simulink model "gm_fil_videosharp_sim"  (R2019a)
settings: Solver=FixedStepDiscrete  StartTime=0.0  StopTime=0.21  RelTol=1e-3
InitFcn:
  | filter = fi(fspecial('unsharp'),1,16,12);
  | 
  | % video size excluding the blanking periods
  | fileName = get_param('fil_videosharp_sim/From Multimedia File',  'inputFilename');
  | x=mmfileinfo(fileName);
  | v = x.Video ;
  | H = v.Height;
  | W = v.Width;
  | %H = 176;
  | %W = 240;
  | activeVideoSize = [H W];
  | 
  | % horizontal and vertical blanking
  | hBlanking = 0;
  | vBlanking = 0;
undefined symbols (not defined in the file or in its folder): fspecial, gcbh, NumBits1, NumBits2, Rec, SDTV, Slope1, Slope2
libraries: simulink x19, visionconversions x3, dspsigattribs x3, dspbuff3 x3, hdlsllib x3, visionsinks x1, dspvision x1, simulink_need_slupdate x1
(part 1 of 3)
settings Model: FPTRunName=Active  SimulationMode=accelerator  ExtModeAutoUpdateStatusClock=off  Creator=wjachimc  LastModifiedBy=rbhar
settings DataIOCC: LimitDataPoints=on  SaveFormat=Structure  SignalLoggingSaveFormat=ModelDataLogs  SaveOutput=off  InspectSignalLogs=on  SaveTime=off  ReturnWorkspaceOutputs=off
settings OptimizationCC: BlockReduction=off  ConditionallyExecuteInputs=off  ExpressionDepthLimit=2147483647  InitFltsAndDblsToZero=on  EfficientMapNaN2IntZero=off  LifeSpan=inf
settings DebuggingCC: UnderspecifiedInitializationDetection=Classic  MergeDetectMultiDrivingBlocksExec=none  InheritedTsInSrcMsg=none  SingleTaskRateTransMsg=error  IntegerOverflowMsg=none  FcnCallInpInsideContextMsg=warning  StateNameClashWarn=warning  PregeneratedLibrarySubsystemCodeDiagnostic=none  SFUnexpectedBacktrackingDiag=warning  SFNoUnconditionalDefaultTransitionDiag=warning  SFExecutionAtInitializationDiag=none  IntegerSaturationMsg=none  ArithmeticOperatorsInVariantConditions=warning
settings HardwareCC: ProdBitPerPointer=32  ProdBitPerSizeT=32  ProdBitPerPtrDiffT=32  ProdLargestAtomicFloat=None  ProdIntDivRoundTo=Undefined  ProdEndianess=Unspecified  ProdWordSize=32  ProdHWDeviceType=ASIC/FPGA->ASIC/FPGA  TargetBitPerPointer=64  TargetBitPerSizeT=64  TargetBitPerPtrDiffT=64  TargetLongLongMode=on  TargetIntDivRoundTo=Zero  TargetEndianess=LittleEndian  TargetWordSize=64  TargetHWDeviceType=MATLAB Host  ProdEqTarget=off
settings ModelReferenceCC: PropagateSignalLabelsOutOfModel=off
settings SFSimCC: SimUseLocalCustomCode=off  SimParseCustomCode=off
settings RTWCC: RTWUseLocalCustomCode=off
settings CodeAppCC: StateflowObjectComments=on
settings GRTTargetCC: TargetLangStandard=C89/C90 (ANSI)  GeneratePreprocessorConditionals=Disable all  CombineOutputUpdateFcns=off  GRTInterface=on
settings ConfigComp: CovMetricSettings=dw  CovHtmlReporting=on  CovSaveCumulativeToWorkspaceVar=on  CovSaveSingleToWorkspaceVar=on  CovExternalEMLEnable=off

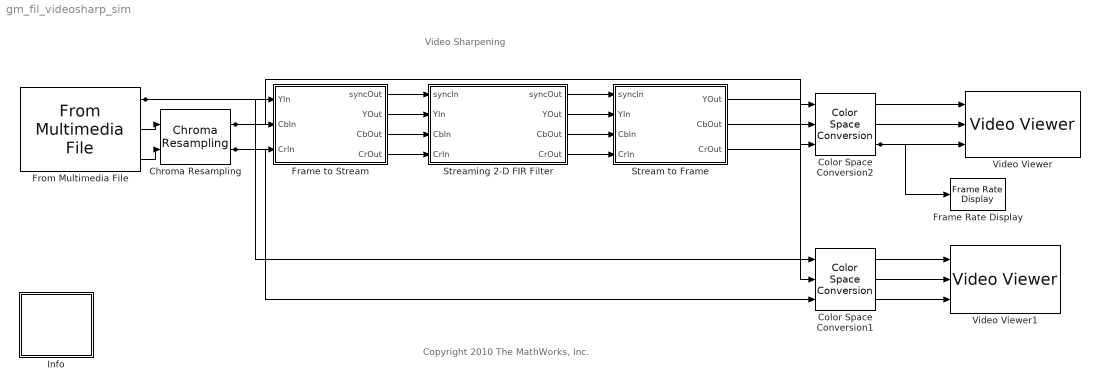
== system gm_fil_videosharp_sim ==
  note: Copyright 2010 The MathWorks, Inc.
  note: Video Sharpening
  Chroma Resampling : visionconversions/Chroma Resampling  resampling=4:2:2 to 4:4:4  interpolation=linear  antialiasing=Default  hcoeff=[0.2 0.6 0.2]  vcoeff=[0.5 0.5]  isInputTransposed=off
      settings: SourceProductName=Computer Vision System Toolbox  SourceProductBaseCode=VP
  Color Space Conversion1 : visionconversions/Color Space  Conversion  conversion=Obsolete  conversionActive=Y'CbCr to R'G'B'  wp_str=D65  rec=Rec. 601 (SDTV)  sys=1125/60/2:1  imagePorts=Separate color signals
      settings: SourceProductName=Computer Vision System Toolbox
  Color Space Conversion2 : visionconversions/Color Space  Conversion  conversion=Obsolete  conversionActive=Y'CbCr to R'G'B'  wp_str=D65  rec=Rec. 601 (SDTV)  sys=1125/60/2:1  imagePorts=Separate color signals
      settings: SourceProductName=Computer Vision System Toolbox
  Frame Rate Display : visionsinks/Frame Rate Display  UpdateRate=3
      settings: SourceProductName=Computer Vision System Toolbox  SourceProductBaseCode=VP
  Frame to Stream : Subsystem  mask(Frame to Stream){hBlanking=hBlanking, vBlanking=vBlanking, isInputRowMajor=off}
      mask prompts: hBlanking "Horizontal blanking:"; vBlanking "Vertical blanking:"; isInputRowMajor "Input image is transposed"
      mask help:
      | This blocks converts a full frame video input into a pixel stream with additional synchronization signals.
      |
      | The specified amount, in pixels, of horizontal blanking is prepended to the left of the video frame while the amount of vertical blanking is appended to the bottom of the video frame.
      mask Display: disp(sprintf('%s\n%s','Frame to', 'Stream'));
  From Multimedia File : dspvision/From Multimedia File  inputFilename=fil_cat.avi  readRange=[1 Inf]  loop=on  numPlays=inf  outputStreams=Video only  videoDataType=uint8  audioDataType=int16  inheritSampleTime=on  userDefinedSampleTime=1  noAudioOutput=off  isIntensityVideo=off  fourcc=YCbCr 4:2:2  colorVideoFormat=Separate color signals  outputEOF=off  dataOrg=Column-major  audioFrameSize=1838  computeAudioFrameSize=off  outSamplingMode=Frame based
      settings: SourceProductBaseCode=VP
  Info : Subsystem  mask(Info){}
      settings: OpenFcn=showdemo('fil_videosharp_sim');
      mask Display: image(imread('fil_demo_info.bmp','bmp'))
  Stream to Frame : Subsystem  mask(Stream to Frame){frameSize=activeVideoSize}
      mask prompts: frameSize "Frame size"
      mask help: Converts stream of pixels into a full frame video based on the corresponding synchronization signals.
      mask Display: disp(sprintf('%s\n%s', 'Stream to', 'Frame'));
  Streaming 2-D FIR Filter : Subsystem  mask(Streaming 2-D FIR Filter){frame_size=activeVideoSize, FILTCOEFF=fi(fspecial('gaussian',[3,3],0.5), 1, 16, 12), PADDING=Replicate, PADVAL=0}
      mask prompts: frame_size "Frame size:"; FILTCOEFF "Filter Coefficient:"; PADDING "Padding Options"; PADVAL "Constant value for padding:"
      mask help: 2-D FIR suitable for FPGA .
      mask init:
      | blkh=gcbh;
      | main_blk = [get(blkh, 'parent'), '/', get(blkh, 'name')];
      | sub_blk = [main_blk, '/', 'Make Neighborhood'];
      | main_value = get_param(main_blk,'PADDING');
      | set_param(sub_blk,'PADDING',main_value);
      | 
      | main_value = get_param(main_blk,'PADVAL');
      | set_param(sub_blk,'PADVAL',main_value);
      mask TypeOptions PADDING: Constant | Replicate | Symmetric
      mask Callback PADDING:
      | maskStr = get_param(gcb,'MaskValues');
      | maskvisi = get_param(gcb,'MaskVisibilities');
      | maskenebles = get_param(gcb,'MaskEnables');
      | if (strcmp(maskStr{3},'Constant') )
      |     maskvisi{4,1}='on';
      | else
      |     maskvisi{4,1}='off';
      | end
      | set_param(gcb,'MaskValues',maskStr);
      | set_param(gcb,'MaskVisibilities',maskvisi);
      | set_param(gcb,'MaskEnables',maskenebles)
      mask Display: disp(sprintf('%s\n%s', 'Streaming', '2-D FIR Filter'));
  Video Viewer : VideoViewer  imagePorts=separate color signals  FigPos=[435 661 410 300]
  Video Viewer1 : VideoViewer  imagePorts=separate color signals  FigPos=[436 659 408 297]
  wires:
  Streaming 2-D FIR Filter/4(CrOut) -> Stream to Frame/4(CrIn)
  Streaming 2-D FIR Filter/3(CbOut) -> Stream to Frame/3(CbIn)
  Frame to Stream/4(CrOut) -> Streaming 2-D FIR Filter/4(CrIn)
  Frame to Stream/3(CbOut) -> Streaming 2-D FIR Filter/3(CbIn)
  Chroma Resampling/2 -> Color Space Conversion1/3, Frame to Stream/3(CrIn)
  Chroma Resampling/1 -> Color Space Conversion1/2, Frame to Stream/2(CbIn)
  From Multimedia File/3 -> Chroma Resampling/2
  From Multimedia File/2 -> Chroma Resampling/1
  Color Space Conversion1/3 -> Video Viewer1/3
  Color Space Conversion1/2 -> Video Viewer1/2
  Color Space Conversion1/1 -> Video Viewer1/1
  Stream to Frame/3(CrOut) -> Color Space Conversion2/3
  Stream to Frame/2(CbOut) -> Color Space Conversion2/2
  Stream to Frame/1(YOut) -> Color Space Conversion2/1
  Color Space Conversion2/3 -> Video Viewer/3, Frame Rate Display/1
  Color Space Conversion2/2 -> Video Viewer/2
  Color Space Conversion2/1 -> Video Viewer/1
  Frame to Stream/2(YOut) -> Streaming 2-D FIR Filter/2(YIn)
  Frame to Stream/1(syncOut) -> Streaming 2-D FIR Filter/1(syncIn)
  Streaming 2-D FIR Filter/2(YOut) -> Stream to Frame/2(YIn)
  Streaming 2-D FIR Filter/1(syncOut) -> Stream to Frame/1(syncIn)
  From Multimedia File/1 -> Color Space Conversion1/1, Frame to Stream/1(YIn)

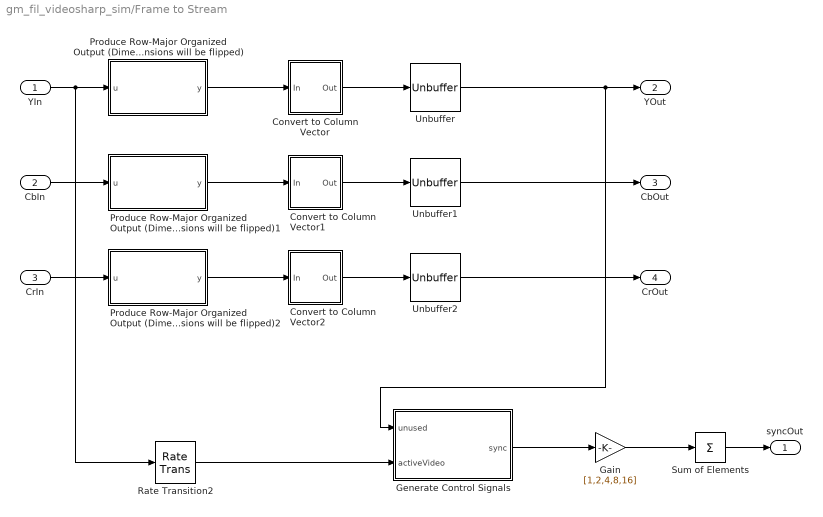
== system gm_fil_videosharp_sim/Frame to Stream ==
  YIn : Inport
  CbIn : Inport  Port=2
  CrIn : Inport  Port=3
  Convert to Column Vector : Subsystem
  Convert to Column Vector1 : Subsystem
  Convert to Column Vector2 : Subsystem
  Gain : Gain  Gain=[1,2,4,8,16]  ParamDataTypeStr=fixdt(0,5,0)  OutDataTypeStr=fixdt(0,5,0)
  Generate Control Signals : MATLAB Function  TreatAsAtomicUnit=on
  Produce Row-Major Organized Output (Dimensions will be flipped) : MATLAB Function  TreatAsAtomicUnit=on
  Produce Row-Major Organized Output (Dimensions will be flipped)1 : MATLAB Function  TreatAsAtomicUnit=on
  Produce Row-Major Organized Output (Dimensions will be flipped)2 : MATLAB Function  TreatAsAtomicUnit=on
  Rate Transition2 : RateTransition  Deterministic=off
  Sum of Elements : Sum  Inputs=+  OutDataTypeStr=fixdt(0,5,0)
  Unbuffer : Unbuffer
      settings: AttributesFormatString="Convert to  Pixel Stream"
  Unbuffer1 : Unbuffer
      settings: AttributesFormatString="Convert to  Pixel Stream"
  Unbuffer2 : Unbuffer
      settings: AttributesFormatString="Convert to  Pixel Stream"
  syncOut : Outport
  YOut : Outport  Port=2
  CbOut : Outport  Port=3
  CrOut : Outport  Port=4
  wires:
  Sum of Elements/1 -> syncOut/1
  Gain/1 -> Sum of Elements/1
  Produce Row-Major Organized Output (Dimensions will be flipped)2/1(y) -> Convert to Column Vector2/1(In)
  Produce Row-Major Organized Output (Dimensions will be flipped)1/1(y) -> Convert to Column Vector1/1(In)
  Produce Row-Major Organized Output (Dimensions will be flipped)/1(y) -> Convert to Column Vector/1(In)
  Unbuffer2/1 -> CrOut/1
  Unbuffer1/1 -> CbOut/1
  CrIn/1 -> Produce Row-Major Organized Output (Dimensions will be flipped)2/1(u)
  CbIn/1 -> Produce Row-Major Organized Output (Dimensions will be flipped)1/1(u)
  Convert to Column Vector2/1(Out) -> Unbuffer2/1
  Convert to Column Vector1/1(Out) -> Unbuffer1/1
  Generate Control Signals/1(sync) -> Gain/1
  Rate Transition2/1 -> Generate Control Signals/2(activeVideo)
  YIn/1 -> Produce Row-Major Organized Output (Dimensions will be flipped)/1(u), Rate Transition2/1
  Unbuffer/1 -> YOut/1, Generate Control Signals/1(unused)
  Convert to Column Vector/1(Out) -> Unbuffer/1

== system gm_fil_videosharp_sim/Info ==

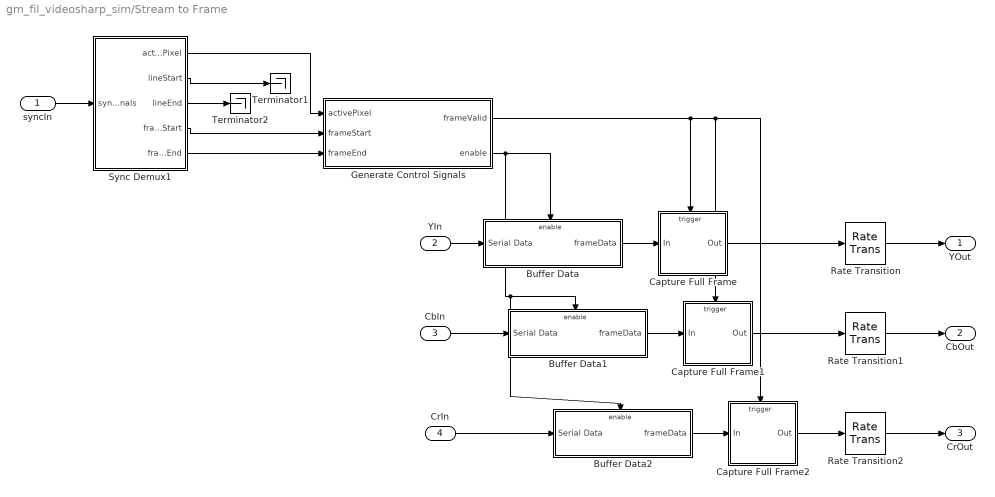
== system gm_fil_videosharp_sim/Stream to Frame ==
  syncIn : Inport
  YIn : Inport  Port=2
  CbIn : Inport  Port=3
  CrIn : Inport  Port=4
  Buffer Data : Subsystem  TreatAsAtomicUnit=on
  Buffer Data1 : Subsystem  TreatAsAtomicUnit=on
  Buffer Data2 : Subsystem  TreatAsAtomicUnit=on
  Capture Full Frame : Subsystem
  Capture Full Frame1 : Subsystem
  Capture Full Frame2 : Subsystem
  Generate Control Signals : MATLAB Function  TreatAsAtomicUnit=on
  Rate Transition : RateTransition  OutPortSampleTime=1/24
  Rate Transition1 : RateTransition  OutPortSampleTime=1/24
  Rate Transition2 : RateTransition  OutPortSampleTime=1/24
  Sync Demux1 : Subsystem
  Terminator1 : Terminator
  Terminator2 : Terminator
  YOut : Outport
  CbOut : Outport  Port=2
  CrOut : Outport  Port=3
  wires:
  Rate Transition2/1 -> CrOut/1
  Rate Transition1/1 -> CbOut/1
  Rate Transition/1 -> YOut/1
  Sync Demux1/5(frameEnd) -> Generate Control Signals/3(frameEnd)
  CrIn/1 -> Buffer Data2/1(Serial Data)
  Capture Full Frame2/1(Out) -> Rate Transition2/1
  Buffer Data2/1(frameData) -> Capture Full Frame2/1(In)
  CbIn/1 -> Buffer Data1/1(Serial Data)
  Capture Full Frame1/1(Out) -> Rate Transition1/1
  Buffer Data1/1(frameData) -> Capture Full Frame1/1(In)
  Sync Demux1/4(frameStart) -> Generate Control Signals/2(frameStart)
  Sync Demux1/1(activePixel) -> Generate Control Signals/1(activePixel)
  Sync Demux1/3(lineEnd) -> Terminator2/1
  Sync Demux1/2(lineStart) -> Terminator1/1
  syncIn/1 -> Sync Demux1/1(syncSignals)
  YIn/1 -> Buffer Data/1(Serial Data)
  Capture Full Frame/1(Out) -> Rate Transition/1
  Buffer Data/1(frameData) -> Capture Full Frame/1(In)
  Generate Control Signals/1(frameValid) -> Capture Full Frame2/Trigger, Capture Full Frame1/Trigger, Capture Full Frame/Trigger
  Generate Control Signals/2(enable) -> Buffer Data2/Enable, Buffer Data1/Enable, Buffer Data/Enable

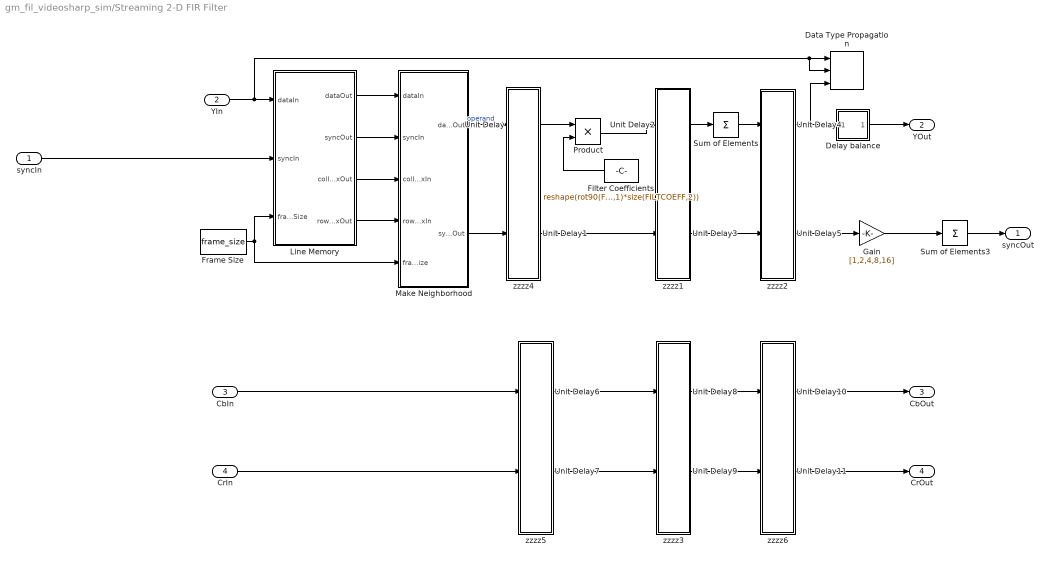
== system gm_fil_videosharp_sim/Streaming 2-D FIR Filter ==
  syncIn : Inport
  YIn : Inport  Port=2
  CbIn : Inport  Port=3
  CrIn : Inport  Port=4
  Data Type Propagation : simulink/Signal Attributes/Data Type Propagation  PropDataType=fixdt(1, 16)  IfRefDouble=double  IfRefSingle=single  IsSigned=IsSigned1 or IsSigned2  NumBitsBase=max([NumBits1 NumBits2])  NumBitsMult=1  NumBitsAdd=0  NumBitsAllowFinal=1:128  PropScaling=2^-10  ValuesUsedBestPrec=[5 -7]  SlopeBase=min([Slope1 Slope2])  SlopeMult=1  SlopeAdd=0  BiasBase=Bias1  BiasMult=1  BiasAdd=0
      settings: SourceProductName=Simulink  SourceProductBaseCode=SL
  Delay balance : Subsystem
  Filter Coefficients : Constant  Value=reshape(rot90(FILTCOEFF,2),1,size(FILTCOEFF,1)*size(FILTCOEFF,2))
  Frame Size : Constant  Value=frame_size  OutDataTypeStr=uint16
  Gain : Gain  Gain=[1,2,4,8,16]  ParamDataTypeStr=fixdt(0,5,0)  OutDataTypeStr=fixdt(0,5,0)
  Line Memory : Subsystem  mask(Line Memory){maxnc=frame_size(2), maxnr=frame_size(1), nL=size(FILTCOEFF,1)}
      mask prompts: maxnc "maximum number of columns in input data"; maxnr "maximum number of rows in input data"; nL "number of lines at the output"
      mask help: Produces Mx1 neighborhood of pixels where M is number of lines.
  Make Neighborhood : Subsystem  mask(Make Neighborhood){NH_ROWS=size(FILTCOEFF,1), NH_COLS=size(FILTCOEFF,2), PADDING=Replicate, PADVAL=0, debug_mode=off, OUTFORMAT=Vector, RIDXWL=ceil(log2(frame_size(1)+1))+1}
      mask prompts: NH_ROWS "number of rows in neighbourhood"; NH_COLS "number of columns in neighbourhood"; PADVAL "value for const padding"; debug_mode "debug mode"; OUTFORMAT "Matrix output"; RIDXWL "row index register wordlength"
      mask help: Creates neighborhood.
      mask TypeOptions PADDING: Constant | Replicate | Symmetric
      mask Callback PADDING:
      | maskStr = get_param(gcb,'MaskValues');
      | maskvisi = get_param(gcb,'MaskVisibilities');
      | maskenebles = get_param(gcb,'MaskEnables');
      | if (strcmp(maskStr{3},'Constant') )
      |     maskvisi{4,1}='on';
      | else
      |     maskvisi{4,1}='off';
      | end
      | set_param(gcb,'MaskValues',maskStr);
      | set_param(gcb,'MaskVisibilities',maskvisi);
      | set_param(gcb,'MaskEnables',maskenebles)
      mask TypeOptions OUTFORMAT: Vector | Matrix
  Product : Product  SaturateOnIntegerOverflow=on
  Sum of Elements : Sum  Inputs=+  OutDataTypeStr=Inherit: Inherit via back propagation  SaturateOnIntegerOverflow=on
  Sum of Elements3 : Sum  Inputs=+  OutDataTypeStr=fixdt(0,5,0)
  Unit Delay{,1..11} (12 alike) : UnitDelay  SampleTime=-1  HasFrameUpgradeWarning=on
  zzzz1 : Subsystem
      settings: AttributesFormatString=|
      | Additional pipeline stage
      | for speed increase
      mask Display: disp('')
  zzzz2 : Subsystem
      settings: AttributesFormatString=|
      | Additional pipeline stage
      | for speed increase
      mask Display: disp('')
  zzzz3 : Subsystem
      settings: AttributesFormatString=|
      | Additional pipeline stage
      | for speed increase
      mask Display: disp('')
  zzzz4 : Subsystem
      settings: AttributesFormatString=|
      | Additional pipeline stage
      | for speed increase
      mask Display: disp('')
  zzzz5 : Subsystem
      settings: AttributesFormatString=|
      | Additional pipeline stage
      | for speed increase
      mask Display: disp('')
  zzzz6 : Subsystem
      settings: AttributesFormatString=|
      | Additional pipeline stage
      | for speed increase
      mask Display: disp('')
  syncOut : Outport
  YOut : Outport  Port=2
  CbOut : Outport  Port=3
  CrOut : Outport  Port=4
  wires:
  Unit Delay11/1 -> CrOut/1
  Unit Delay10/1 -> CbOut/1
  Unit Delay9/1 -> Unit Delay11/1
  Unit Delay8/1 -> Unit Delay10/1
  Unit Delay7/1 -> Unit Delay9/1
  Unit Delay6/1 -> Unit Delay8/1
  CrIn/1 -> Unit Delay7/1
  CbIn/1 -> Unit Delay6/1
  Unit Delay5/1 -> Gain/1
  Sum of Elements3/1 -> syncOut/1
  Gain/1 -> Sum of Elements3/1
  Delay balance/1(Out1) -> YOut/1
  Frame Size/1 -> Make Neighborhood/5(frameSize), Line Memory/3(frameSize)
  Sum of Elements/1 -> Unit Delay4/1
  YIn/1 -> Line Memory/1(dataIn), Data Type Propagation/2, Data Type Propagation/1
  Make Neighborhood/1(dataOut) -> Unit Delay/1  "operand"
  syncIn/1 -> Line Memory/2(syncIn)
  Product/1 -> Unit Delay2/1
  Line Memory/1(dataOut) -> Make Neighborhood/1(dataIn)
  Line Memory/2(syncOut) -> Make Neighborhood/2(syncIn)
  Line Memory/3(colIndexOut) -> Make Neighborhood/3(colIndexIn)
  Line Memory/4(rowIndexOut) -> Make Neighborhood/4(rowIndexIn)
  Unit Delay/1 -> Product/1
  Unit Delay1/1 -> Unit Delay3/1
  Unit Delay2/1 -> Sum of Elements/1
  Unit Delay3/1 -> Unit Delay5/1
  Make Neighborhood/2(syncOut) -> Unit Delay1/1
  Filter Coefficients/1 -> Product/2
  Unit Delay4/1 -> Delay balance/1(In1), Data Type Propagation/3

== system gm_fil_videosharp_sim/Frame to Stream/Convert to Column Vector ==
  In : Inport
  Balance Latencies : Delay  DelayLength=uint8(strcmpi(get_param(bdroot(gcbh),'SolverMode'), 'SingleTasking'))  InitialCondition=0  UseCircularBuffer=on
  Convert 2-D to 1-D : dspsigattribs/Convert 2-D to 1-D
      settings: SourceProductName=DSP System Toolbox  SourceProductBaseCode=DS
  Frame Conversion : FrameConversion
  Out : Outport
  wires:
  Frame Conversion/1 -> Out/1
  In/1 -> Balance Latencies/1
  Balance Latencies/1 -> Convert 2-D to 1-D/1
  Convert 2-D to 1-D/1 -> Frame Conversion/1

== system gm_fil_videosharp_sim/Frame to Stream/Convert to Column Vector1 ==
  In : Inport
  Balance Latencies : Delay  DelayLength=uint8(strcmpi(get_param(bdroot(gcbh),'SolverMode'), 'SingleTasking'))  InitialCondition=0  UseCircularBuffer=on
  Convert 2-D to 1-D : dspsigattribs/Convert 2-D to 1-D
      settings: SourceProductName=DSP System Toolbox  SourceProductBaseCode=DS
  Frame Conversion : FrameConversion
  Out : Outport
  wires:
  Convert 2-D to 1-D/1 -> Frame Conversion/1
  Balance Latencies/1 -> Convert 2-D to 1-D/1
  In/1 -> Balance Latencies/1
  Frame Conversion/1 -> Out/1

== system gm_fil_videosharp_sim/Frame to Stream/Convert to Column Vector2 ==
  In : Inport
  Balance Latencies : Delay  DelayLength=uint8(strcmpi(get_param(bdroot(gcbh),'SolverMode'), 'SingleTasking'))  InitialCondition=0  UseCircularBuffer=on
  Convert 2-D to 1-D : dspsigattribs/Convert 2-D to 1-D
      settings: SourceProductName=DSP System Toolbox  SourceProductBaseCode=DS
  Frame Conversion : FrameConversion
  Out : Outport
  wires:
  Frame Conversion/1 -> Out/1
  In/1 -> Balance Latencies/1
  Balance Latencies/1 -> Convert 2-D to 1-D/1
  Convert 2-D to 1-D/1 -> Frame Conversion/1

== system gm_fil_videosharp_sim/Stream to Frame/Buffer Data ==
  Serial Data : Inport
  Enable : EnablePort  PropagateVarSize=During execution
  Delay Line : dspbuff3/Delay Line  siz=prod(frameSize)  ic=0  directfeed=off  enable_output=off  hold_output=off  OutputFrames=on
      settings: SourceProductName=DSP System Toolbox  SourceProductBaseCode=DS
  Frame Conversion : FrameConversion  OutFrame=Sample-based
  frameData : Outport
  wires:
  Frame Conversion/1 -> frameData/1
  Serial Data/1 -> Delay Line/1
  Delay Line/1 -> Frame Conversion/1

== system gm_fil_videosharp_sim/Stream to Frame/Buffer Data1 ==
  Serial Data : Inport
  Enable : EnablePort  PropagateVarSize=During execution
  Delay Line : dspbuff3/Delay Line  siz=prod(frameSize)  ic=0  directfeed=off  enable_output=off  hold_output=off  OutputFrames=on
      settings: SourceProductName=DSP System Toolbox  SourceProductBaseCode=DS
  Frame Conversion : FrameConversion  OutFrame=Sample-based
  frameData : Outport
  wires:
  Delay Line/1 -> Frame Conversion/1
  Serial Data/1 -> Delay Line/1
  Frame Conversion/1 -> frameData/1

== system gm_fil_videosharp_sim/Stream to Frame/Buffer Data2 ==
  Serial Data : Inport
  Enable : EnablePort  PropagateVarSize=During execution
  Delay Line : dspbuff3/Delay Line  siz=prod(frameSize)  ic=0  directfeed=off  enable_output=off  hold_output=off  OutputFrames=on
      settings: SourceProductName=DSP System Toolbox  SourceProductBaseCode=DS
  Frame Conversion : FrameConversion  OutFrame=Sample-based
  frameData : Outport
  wires:
  Frame Conversion/1 -> frameData/1
  Serial Data/1 -> Delay Line/1
  Delay Line/1 -> Frame Conversion/1

== system gm_fil_videosharp_sim/Stream to Frame/Capture Full Frame ==
  note: Get back to col-major
  In : Inport
  Trigger : TriggerPort  VariantControl=(inherit)
  Permute Dimensions : PermuteDimensions
  Reshape : Reshape  OutputDimensionality=Customize  OutputDimensions=fliplr(frameSize)
  Out : Outport
  wires:
  In/1 -> Reshape/1
  Reshape/1 -> Permute Dimensions/1
  Permute Dimensions/1 -> Out/1

== system gm_fil_videosharp_sim/Stream to Frame/Capture Full Frame1 ==
  note: Get back to col-major
  In : Inport
  Trigger : TriggerPort  VariantControl=(inherit)
  Permute Dimensions : PermuteDimensions
  Reshape : Reshape  OutputDimensionality=Customize  OutputDimensions=fliplr(frameSize)
  Out : Outport
  wires:
  Permute Dimensions/1 -> Out/1
  Reshape/1 -> Permute Dimensions/1
  In/1 -> Reshape/1

== system gm_fil_videosharp_sim/Stream to Frame/Capture Full Frame2 ==
  note: Get back to col-major
  In : Inport
  Trigger : TriggerPort  VariantControl=(inherit)
  Permute Dimensions : PermuteDimensions
  Reshape : Reshape  OutputDimensionality=Customize  OutputDimensions=fliplr(frameSize)
  Out : Outport
  wires:
  In/1 -> Reshape/1
  Reshape/1 -> Permute Dimensions/1
  Permute Dimensions/1 -> Out/1

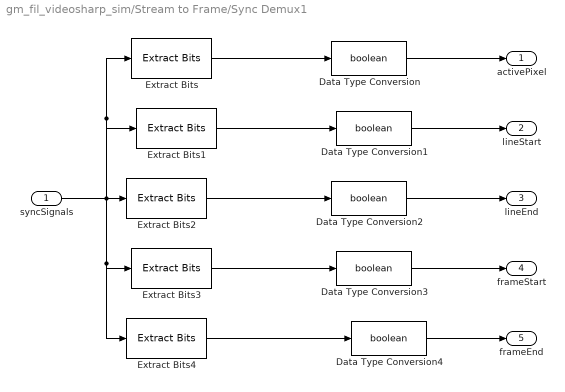
== system gm_fil_videosharp_sim/Stream to Frame/Sync Demux1 ==
  syncSignals : Inport
  Data Type Conversion{,1..4} (5 alike) : DataTypeConversion  OutDataTypeStr=boolean
  Extract Bits : simulink/Logic and Bit Operations/Extract Bits  bitsToExtract=Range of bits  numBits=8  bitIdxRange=[0]  outScalingMode=Treat bit field as an integer
      settings: SourceProductName=Simulink
  Extract Bits1 : simulink/Logic and Bit Operations/Extract Bits  bitsToExtract=Range of bits  numBits=8  bitIdxRange=[1]  outScalingMode=Treat bit field as an integer
      settings: SourceProductName=Simulink
  Extract Bits2 : simulink/Logic and Bit Operations/Extract Bits  bitsToExtract=Range of bits  numBits=8  bitIdxRange=[2]  outScalingMode=Treat bit field as an integer
      settings: SourceProductName=Simulink
  Extract Bits3 : simulink/Logic and Bit Operations/Extract Bits  bitsToExtract=Range of bits  numBits=8  bitIdxRange=[3]  outScalingMode=Treat bit field as an integer
      settings: SourceProductName=Simulink
  Extract Bits4 : simulink/Logic and Bit Operations/Extract Bits  bitsToExtract=Range of bits  numBits=8  bitIdxRange=[4]  outScalingMode=Treat bit field as an integer
      settings: SourceProductName=Simulink
  activePixel : Outport
  lineStart : Outport  Port=2
  lineEnd : Outport  Port=3
  frameStart : Outport  Port=4
  frameEnd : Outport  Port=5
  wires:
  Data Type Conversion4/1 -> frameEnd/1
  Data Type Conversion3/1 -> frameStart/1
  Data Type Conversion2/1 -> lineEnd/1
  Data Type Conversion1/1 -> lineStart/1
  Data Type Conversion/1 -> activePixel/1
  Extract Bits/1 -> Data Type Conversion/1
  Extract Bits1/1 -> Data Type Conversion1/1
  Extract Bits2/1 -> Data Type Conversion2/1
  Extract Bits3/1 -> Data Type Conversion3/1
  Extract Bits4/1 -> Data Type Conversion4/1
  syncSignals/1 -> Extract Bits4/1, Extract Bits3/1, Extract Bits2/1, Extract Bits1/1, Extract Bits/1

== system gm_fil_videosharp_sim/Streaming 2-D FIR Filter/Delay balance ==
  In1 : Inport
  Add : Sum  OutDataTypeStr=Inherit: Inherit via back propagation
  Constant : Constant  OutDataTypeStr=boolean
  Constant1 : Constant  Value=2^ceil(log2(H*W))-(W*(H-4)-9)  OutDataTypeStr=Inherit: Inherit via back propagation
  Counter Limited : simulink/Sources/Counter Limited  uplimit=2^ceil(log2(H*W))-1  tsamp=-1
  Counter Limited1 : simulink/Sources/Counter Limited  uplimit=2^ceil(log2(H*W))-1  tsamp=-1
  Data Type Conversion : DataTypeConversion
  Simple Dual Port RAM : hdlsllib/HDL RAMs/Simple Dual Port RAM  ram_size=ceil(log2(H*W))
      settings: SourceProductName=HDL Coder  SourceProductBaseCode=HD
  Out1 : Outport
  wires:
  Constant/1 -> Simple Dual Port RAM/3
  Counter Limited/1 -> Data Type Conversion/1
  Simple Dual Port RAM/1 -> Out1/1
  In1/1 -> Simple Dual Port RAM/1
  Counter Limited1/1 -> Add/1
  Add/1 -> Simple Dual Port RAM/4
  Constant1/1 -> Add/2
  Data Type Conversion/1 -> Simple Dual Port RAM/2

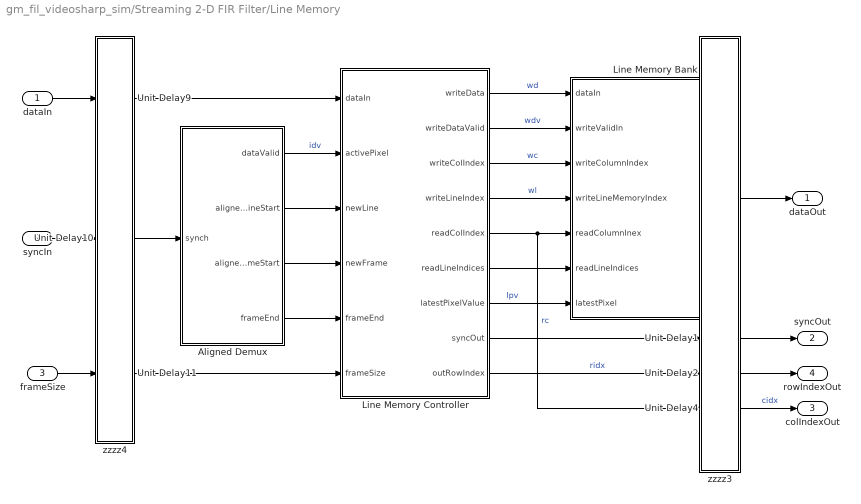
== system gm_fil_videosharp_sim/Streaming 2-D FIR Filter/Line Memory ==
  dataIn : Inport
  syncIn : Inport  Port=2
  frameSize : Inport  Port=3
  Aligned Demux : Subsystem
  Line Memory Bank : Subsystem
  Line Memory Controller : Subsystem
  Unit Delay{1..2,4,9..11} (6 alike) : UnitDelay  SampleTime=-1  HasFrameUpgradeWarning=on
  zzzz3 : Subsystem
      settings: AttributesFormatString=Delay balancing
      mask Display: disp('')
  zzzz4 : Subsystem
      settings: AttributesFormatString=|
      | Additional pipeline stage
      | for speed increase
      mask Display: disp('')
  dataOut : Outport
  syncOut : Outport  Port=2
  colIndexOut : Outport  Port=3
  rowIndexOut : Outport  Port=4
  wires:
  Line Memory Controller/1(writeData) -> Line Memory Bank/1(dataIn)  "wd"
  dataIn/1 -> Unit Delay9/1
  Line Memory Bank/1(dataOut) -> dataOut/1
  Line Memory Controller/2(writeDataValid) -> Line Memory Bank/2(writeValidIn)  "wdv"
  syncIn/1 -> Unit Delay10/1
  Unit Delay10/1 -> Aligned Demux/1(synch)
  frameSize/1 -> Unit Delay11/1
  Unit Delay11/1 -> Line Memory Controller/6(frameSize)
  Line Memory Controller/3(writeColIndex) -> Line Memory Bank/3(writeColumnIndex)  "wc"
  Line Memory Controller/4(writeLineIndex) -> Line Memory Bank/4(writeLineMemoryIndex)  "wl"
  Line Memory Controller/5(readColIndex) -> Line Memory Bank/5(readColumnInex), Unit Delay4/1  "rc"
  Line Memory Controller/6(readLineIndices) -> Line Memory Bank/6(readLineIndices)
  Unit Delay9/1 -> Line Memory Controller/1(dataIn)
  Aligned Demux/1(dataValid) -> Line Memory Controller/2(activePixel)  "idv"
  Aligned Demux/2(alignedLineStart) -> Line Memory Controller/3(newLine)
  Aligned Demux/3(alignedFrameStart) -> Line Memory Controller/4(newFrame)
  Aligned Demux/4(frameEnd) -> Line Memory Controller/5(frameEnd)
  Line Memory Controller/7(latestPixelValue) -> Line Memory Bank/7(latestPixel)  "lpv"
  Line Memory Controller/9(outRowIndex) -> Unit Delay2/1  "ridx"
  Unit Delay4/1 -> colIndexOut/1  "cidx"
  Unit Delay2/1 -> rowIndexOut/1
  Unit Delay1/1 -> syncOut/1
  Line Memory Controller/8(syncOut) -> Unit Delay1/1

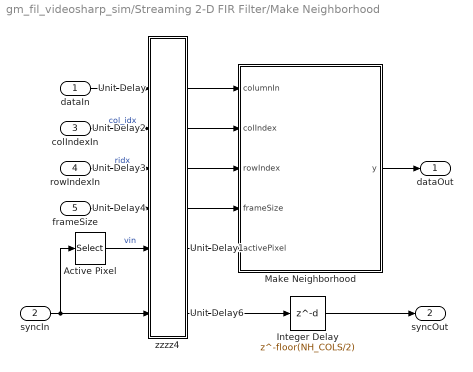
== system gm_fil_videosharp_sim/Streaming 2-D FIR Filter/Make Neighborhood ==
  dataIn : Inport
  syncIn : Inport  Port=2
  colIndexIn : Inport  Port=3
  rowIndexIn : Inport  Port=4
  frameSize : Inport  Port=5
  Active Pixel : Selector  IndexMode=Zero-based  InputPortWidth=5  IndexOptions=Index vector (dialog)  Indices=0  OutputSizes=1
  Integer Delay : Delay  DelayLength=floor(NH_COLS/2)
  Make Neighborhood : MATLAB Function  TreatAsAtomicUnit=on
  Unit Delay{,1..4,6} (6 alike) : UnitDelay  SampleTime=-1  HasFrameUpgradeWarning=on
  zzzz4 : Subsystem
      settings: AttributesFormatString=|
      | Additional pipeline stage
      | for speed increase
      mask Display: disp('')
  dataOut : Outport
  syncOut : Outport  Port=2
  wires:
  Make Neighborhood/1(y) -> dataOut/1
  syncIn/1 -> Unit Delay6/1, Active Pixel/1
  Integer Delay/1 -> syncOut/1
  dataIn/1 -> Unit Delay/1
  Active Pixel/1 -> Unit Delay1/1  "vin"
  colIndexIn/1 -> Unit Delay2/1  "col_idx"
  rowIndexIn/1 -> Unit Delay3/1  "ridx"
  frameSize/1 -> Unit Delay4/1
  Unit Delay6/1 -> Integer Delay/1
  Unit Delay/1 -> Make Neighborhood/1(columnIn)
  Unit Delay1/1 -> Make Neighborhood/5(activePixel)
  Unit Delay2/1 -> Make Neighborhood/2(colIndex)
  Unit Delay3/1 -> Make Neighborhood/3(rowIndex)
  Unit Delay4/1 -> Make Neighborhood/4(frameSize)

== system gm_fil_videosharp_sim/Streaming 2-D FIR Filter/zzzz1 ==

== system gm_fil_videosharp_sim/Streaming 2-D FIR Filter/zzzz2 ==

== system gm_fil_videosharp_sim/Streaming 2-D FIR Filter/zzzz3 ==

== system gm_fil_videosharp_sim/Streaming 2-D FIR Filter/zzzz4 ==

== system gm_fil_videosharp_sim/Streaming 2-D FIR Filter/zzzz5 ==

== system gm_fil_videosharp_sim/Streaming 2-D FIR Filter/zzzz6 ==

== system gm_fil_videosharp_sim/Streaming 2-D FIR Filter/Line Memory/Aligned Demux ==
  synch : Inport
  Aligned Pulse : MATLAB Function  TreatAsAtomicUnit=on
  Aligned Pulse1 : MATLAB Function  TreatAsAtomicUnit=on
  Sync Demux : Subsystem
  Terminator : Terminator
  dataValid : Outport
  alignedLineStart : Outport  Port=2
  alignedFrameStart : Outport  Port=3
  frameEnd : Outport  Port=4
  wires:
  Sync Demux/4(frameStart) -> Aligned Pulse1/2(earlyPulse)
  Sync Demux/2(lineStart) -> Aligned Pulse/2(earlyPulse)
  Sync Demux/5(frameEnd) -> frameEnd/1
  Sync Demux/3(lineEnd) -> Terminator/1
  Sync Demux/1(activePixel) -> Aligned Pulse1/1(valid), Aligned Pulse/1(valid), dataValid/1
  synch/1 -> Sync Demux/1(syncSignals)
  Aligned Pulse/1(alignedPulse) -> alignedLineStart/1
  Aligned Pulse1/1(alignedPulse) -> alignedFrameStart/1

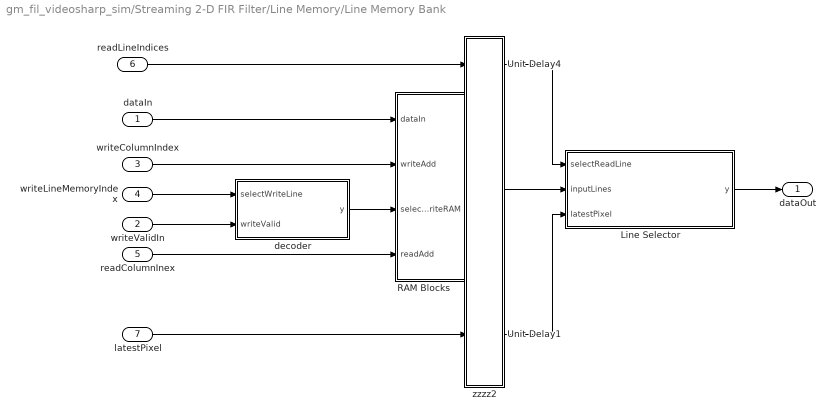
== system gm_fil_videosharp_sim/Streaming 2-D FIR Filter/Line Memory/Line Memory Bank ==
  dataIn : Inport
  writeValidIn : Inport  Port=2
  writeColumnIndex : Inport  Port=3
  writeLineMemoryIndex : Inport  Port=4
  readColumnInex : Inport  Port=5
  readLineIndices : Inport  Port=6
  latestPixel : Inport  Port=7
  Line Selector : MATLAB Function  TreatAsAtomicUnit=on
  "RAM Blocks " : Subsystem  mask{nb=nL-1, WL=ceil(log2(maxnc)), eval_nb=2, eval_WL=8}
      mask prompts: nb "Number of blocks:"; WL "Address port width (2 to 16):"; eval_nb "evaluated nb"; eval_WL "evaluated WL"
      mask init:
      | blk = gcb;
      | set_param(blk,'eval_nb',num2str(nb));
      | set_param(blk,'eval_WL',num2str(WL));
      | 
      | % hws = get_param(bdroot, 'modelworkspace');
      | % hws.assignin('VIPHDL_numb_RAM_block', nb);
      | % hws.assignin('VIPHDL_RAM_block_WL', WL);
  Unit Delay1 : UnitDelay  SampleTime=-1  HasFrameUpgradeWarning=on
  Unit Delay4 : UnitDelay  SampleTime=-1  HasFrameUpgradeWarning=on
  decoder : MATLAB Function  TreatAsAtomicUnit=on
  zzzz2 : Subsystem
      settings: AttributesFormatString=Delay balancing
      mask Display: disp('')
  dataOut : Outport
  wires:
  readLineIndices/1 -> Unit Delay4/1
  Unit Delay4/1 -> Line Selector/1(selectReadLine)
  "RAM Blocks "/1(dataOut) -> Line Selector/2(inputLines)
  dataIn/1 -> "RAM Blocks "/1(dataIn)
  writeColumnIndex/1 -> "RAM Blocks "/2(writeAdd)
  readColumnInex/1 -> "RAM Blocks "/4(readAdd)
  writeLineMemoryIndex/1 -> decoder/1(selectWriteLine)
  decoder/1(y) -> "RAM Blocks "/3(selectWriteRAM)
  Line Selector/1(y) -> dataOut/1
  writeValidIn/1 -> decoder/2(writeValid)
  latestPixel/1 -> Unit Delay1/1
  Unit Delay1/1 -> Line Selector/3(latestPixel)
